simulink subsystem "kinematics_quaternion"  (R2024b)
settings: Solver=VariableStepAuto  StartTime=0.0  StopTime=10.0  RelTol=1e-3
undefined symbols (not defined in the file or in its folder): e0_0, e1_0, e2_0, e3_0, rail_angle
libraries: sharedtransform x1
settings Model: Creator=finnb  LastModifiedBy=finnb

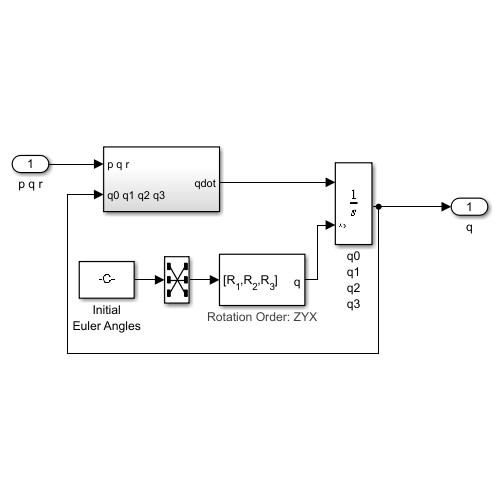
[thumbnail: Simulink's stored preview of the top-level diagram]
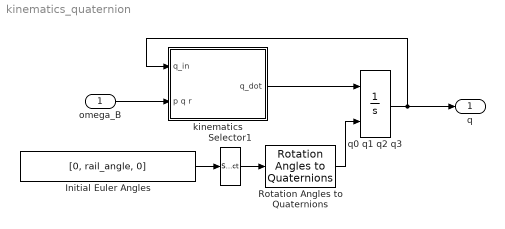
== system kinematics_quaternion ==
  omega_B : Inport  OutDataTypeStr=double
  Initial Euler Angles : Constant  Value=[0, rail_angle, 0]
  Rotation Angles to Quaternions : sharedtransform/Rotation Angles to Quaternions  rotationOrder=ZYX  aMode=aMode
  Selector1 : Selector  InputPortWidth=3  IndexOptions=Index vector (dialog)  Indices=[3 2 1]  OutputSizes=1
  kinematics : Subsystem
  q0 q1 q2 q3 : Integrator  InitialConditionSource=external  InitialCondition=[e0_0 e1_0 e2_0 e3_0]
  q : Outport  OutDataTypeStr=double  VectorParamsAs1DForOutWhenUnconnected=off
  wires:
  q0 q1 q2 q3/1 -> q/1, kinematics/1(q_in)
  Initial Euler Angles/1 -> Selector1/1
  Selector1/1 -> Rotation Angles to Quaternions/1
  kinematics/1(q_dot) -> q0 q1 q2 q3/1
  omega_B/1 -> kinematics/2(p q r)
  Rotation Angles to Quaternions/1 -> q0 q1 q2 q3/2

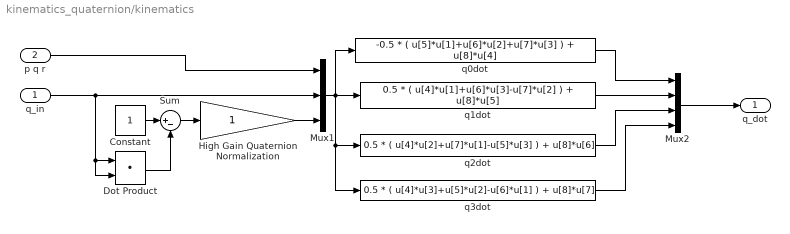
== system kinematics_quaternion/kinematics ==
  q_in : Inport  OutDataTypeStr=double
  p q r : Inport  Port=2  OutDataTypeStr=double
  Constant : Constant
  Dot Product : DotProduct  InputSameDT=off  OutDataTypeStr=Inherit: Inherit via internal rule
  High Gain Quaternion Normalization : Gain  SaturateOnIntegerOverflow=on  OutDataTypeStr=Inherit: Same as input  ParamDataTypeStr=Inherit: Same as input
  Mux1 : Mux  Inputs=[3 4 1]
  Mux2 : Mux
  Sum : Sum  Inputs=|+-  InputSameDT=on  SaturateOnIntegerOverflow=on  OutDataTypeStr=Inherit: Same as first input
  q0dot : Fcn  Expr=-0.5 * ( u[5]*u[1]+u[6]*u[2]+u[7]*u[3] ) + u[8]*u[4]
  q1dot : Fcn  Expr=0.5 * ( u[4]*u[1]+u[6]*u[3]-u[7]*u[2] ) + u[8]*u[5]
  q2dot : Fcn  Expr=0.5 * ( u[4]*u[2]+u[7]*u[1]-u[5]*u[3] ) + u[8]*u[6]
  q3dot : Fcn  Expr=0.5 * ( u[4]*u[3]+u[5]*u[2]-u[6]*u[1] ) + u[8]*u[7]
  q_dot : Outport  OutDataTypeStr=double  VectorParamsAs1DForOutWhenUnconnected=off
  wires:
  Constant/1 -> Sum/1
  q1dot/1 -> Mux2/2
  Mux1/1 -> q2dot/1, q3dot/1, q0dot/1, q1dot/1
  p q r/1 -> Mux1/1
  q0dot/1 -> Mux2/1
  Dot Product/1 -> Sum/2
  q3dot/1 -> Mux2/4
  q2dot/1 -> Mux2/3
  High Gain Quaternion Normalization/1 -> Mux1/3
  q_in/1 -> Dot Product/1, Dot Product/2, Mux1/2
  Mux2/1 -> q_dot/1
  Sum/1 -> High Gain Quaternion Normalization/1
